simulink model "PD_double_pend"  (R2021a)
settings: Solver=FixedStepAuto  StartTime=0.0  StopTime=10  FixedStep=.01  RelTol=1e-3
model workspace (MAT data in the model file):
  exo_pos_cost_10 = param.Continuous
  exo_pos_cost_10.Size_ = [1 1]
  exo_pos_cost_10.Value_ = 1.48511326465
  exo_pos_cost_10.pID = paramid.Variable
  exo_pos_cost_10.pID.Name = 'exo_pos_cost'
values from neighbouring files (symbols this model uses):
  Dm1 = [1000,0;0,103.228187679703]    [no_exo.m]    (also in non_same_length.m = [30,0;0,30]; play_file.m = [30,0;0,30]; play_file22.m = [300,0;0,300]; play_file23.m = [30,0;0,30])
  Km1 = [1000,0;0,1000]    [no_exo.m]    (also in non_same_length.m = [30, 0; 0 30]; play_file.m = [30, 0; 0 30]; play_file22.m = [300, 0; 0 300]; play_file23.m = [30, 0; 0 30])
  l = [0.324, 0.3900]    [myStateTransitionFcn.m]
  lh = [0.324, 0.3900]    [no_exo.m]    (also in non_same_length.m; play_file.m; play_file22.m; play_file23.m)
  mh = [11.824, 3.848]    [no_exo.m]    (also in non_same_length.m; play_file.m; play_file22.m; play_file23.m)
undefined symbols (not defined in the file or in its folder): l1, l2, me2
libraries: robotcorelib x1
settings Model: Creator=nathanielgoldfarb  LastModifiedBy=nathanielgoldfarb
settings SolverCC: AlgebraicLoopSolver=TrustRegion
settings DataIOCC: ReturnWorkspaceOutputsName=SDOSimTest_Log
settings DebuggingCC: SFMachineParentedDataDiag=warning

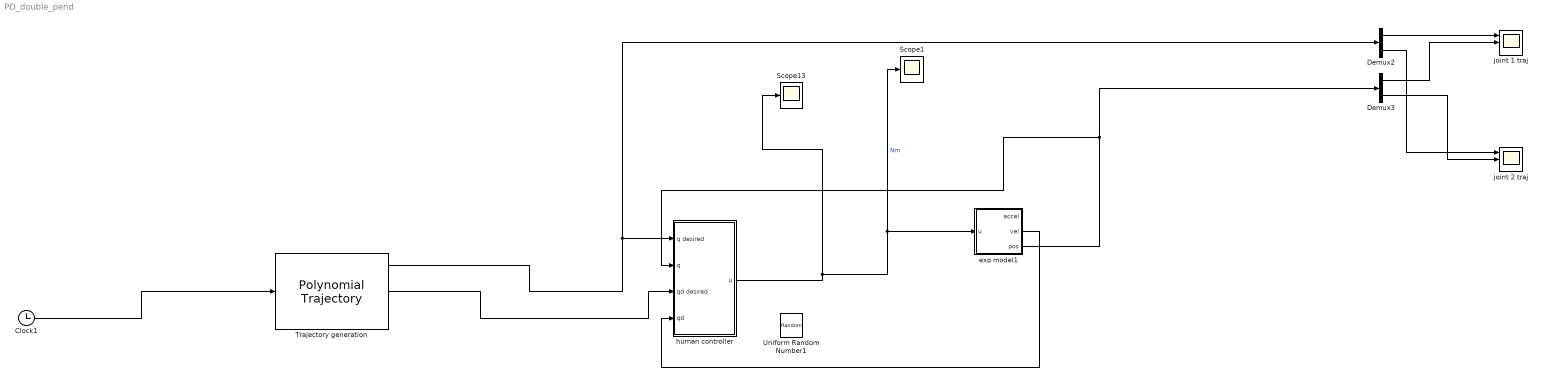
== system PD_double_pend ==
  Clock1 : Clock
  Demux2 : Demux  Outputs=2
  Demux3 : Demux  Outputs=2
  Scope1 : Scope
  Scope13 : Scope
  Trajectory generation : robotcorelib/Polynomial Trajectory  WaypointSource=Internal  Waypoints="[ 0 , -pi, 0;  0 -0.5*pi,0 ]"  TimePoints=[ 0, 5, 10]  TimeInterval=[ 1, 4 ]  Method=Cubic Polynomial  ParameterSource=Internal  VelocityBoundaryCondition=zeros( 2, 3 )  AccelerationBoundaryCondition=zeros( 2, 5 )  SimulateUsing=Interpreted execution
  Uniform Random Number1 : UniformRandomNumber  Minimum=-10  Maximum=10  SampleTime=0.1
  exo model1 : Subsystem
  human controller : Subsystem
  joint 1 traj : Scope  NumInputPorts=3
  joint 2 traj : Scope  NumInputPorts=3
  wires:
  Demux3/1 -> joint 1 traj/2
  Clock1/1 -> Trajectory generation/1
  Demux2/1 -> joint 1 traj/1
  Trajectory generation/1 -> human controller/1(q desired), Demux2/1
  Demux3/2 -> joint 2 traj/2
  Trajectory generation/2 -> human controller/3(qd desired)
  exo model1/3(pos) -> Demux3/1, human controller/2(q)
  exo model1/2(vel) -> human controller/4(qd)
  human controller/1(u) -> exo model1/1(u), Scope1/1, Scope13/1  "Nm"
  Demux2/2 -> joint 2 traj/1

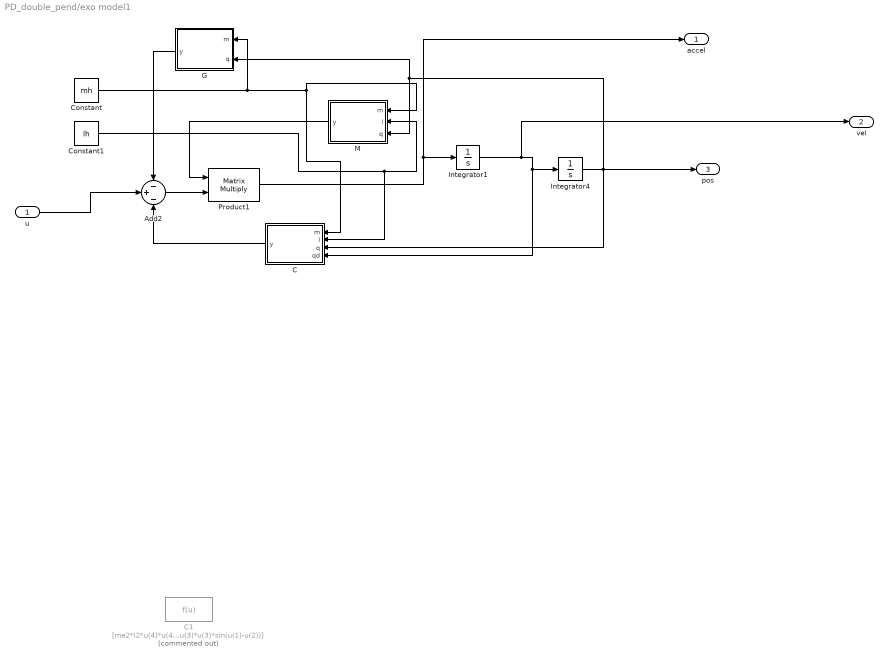
== system PD_double_pend/exo model1 ==
  u : Inport
  Add2 : Sum  Inputs=-+-
  C : MATLAB Function  TreatAsAtomicUnit=on
  C1 : Fcn  Commented=on  Expr=[me2*l2*u(4)*u(4)*sin(u(1)-u(2)); -me2*l1*u(3)*u(3)*sin(u(1)-u(2))]
  Constant : Constant  Value=mh
  Constant1 : Constant  Value=lh
  G : MATLAB Function  TreatAsAtomicUnit=on
  Integrator1 : Integrator  InitialCondition=[0;0]
  Integrator4 : Integrator  InitialCondition=[0.01;0.01]
  M : MATLAB Function  TreatAsAtomicUnit=on
  Product1 : Product  Multiplication=Matrix(*)
  accel : Outport
  vel : Outport  Port=2
  pos : Outport  Port=3
  wires:
  Constant/1 -> G/1(m), M/1(m), C/1(m)
  M/1(y) -> Product1/1
  Add2/1 -> Product1/2
  C/1(y) -> Add2/3
  G/1(y) -> Add2/1
  u/1 -> Add2/2
  Product1/1 -> accel/1, Integrator1/1
  Constant1/1 -> C/2(l), M/2(l)
  Integrator4/1 -> C/3(q), pos/1, M/3(q), G/2(q)
  Integrator1/1 -> vel/1, C/4(qd), Integrator4/1

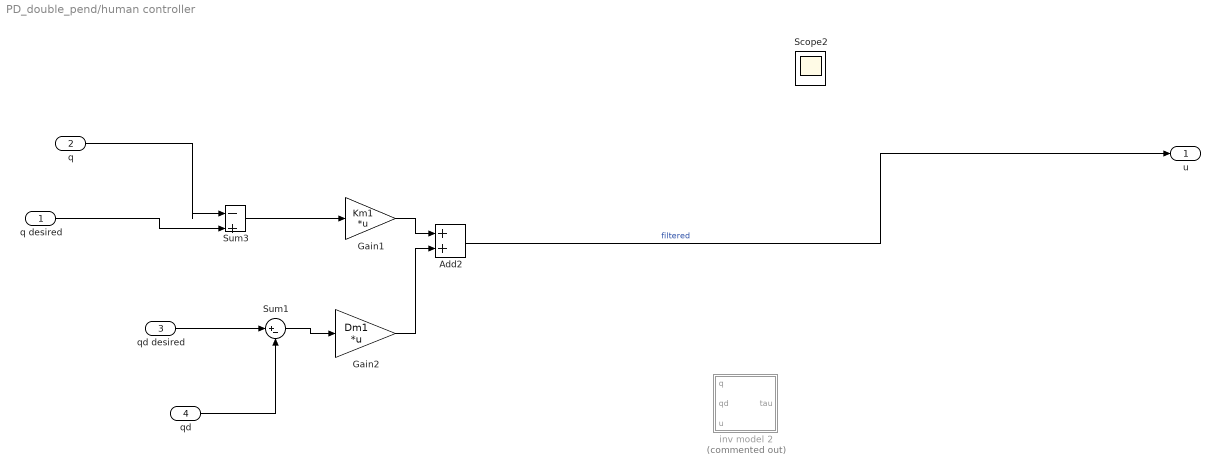
== system PD_double_pend/human controller ==
  q desired : Inport
  q : Inport  Port=2
  qd desired : Inport  Port=3
  qd : Inport  Port=4
  Add2 : Sum
  Gain1 : Gain  Gain=Km1  Multiplication=Matrix(K*u)
  Gain2 : Gain  Gain=Dm1  Multiplication=Matrix(K*u)
  Scope2 : Scope  NumInputPorts=3
  Sum1 : Sum  Inputs=|+-
  Sum3 : Sum  Inputs=|-+
  inv model 2 : Subsystem  Commented=on
  u : Outport
  wires:
  Sum1/1 -> Gain2/1
  qd/1 -> Sum1/2
  Sum3/1 -> Gain1/1
  Gain2/1 -> Add2/2
  q desired/1 -> Sum3/2
  Gain1/1 -> Add2/1
  qd desired/1 -> Sum1/1
  q/1 -> Sum3/1
  Add2/1 -> u/1  "filtered"

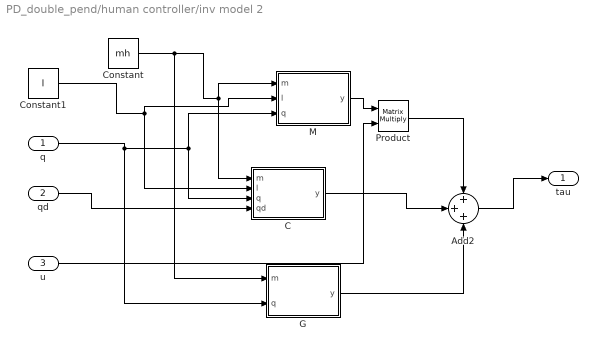
== system PD_double_pend/human controller/inv model 2 ==
  q : Inport
  qd : Inport  Port=2
  "u " : Inport  Port=3
  Add2 : Sum  Inputs=+++
  C : MATLAB Function  TreatAsAtomicUnit=on
  Constant : Constant  Value=mh
  Constant1 : Constant  Value=l
  G : MATLAB Function  TreatAsAtomicUnit=on
  M : MATLAB Function  TreatAsAtomicUnit=on
  Product : Product  Multiplication=Matrix(*)
  "tau " : Outport
  wires:
  Constant1/1 -> C/2(l), M/2(l)
  Constant/1 -> G/1(m), C/1(m), M/1(m)
  "u "/1 -> Product/2
  Product/1 -> Add2/1
  M/1(y) -> Product/1
  qd/1 -> C/4(qd)
  q/1 -> G/2(q), C/3(q), M/3(q)
  Add2/1 -> "tau "/1
  C/1(y) -> Add2/2
  G/1(y) -> Add2/3

== matlab function PD_double_pend/human controller/inv model 2/C ==
  data: m input; l input; q input; y output; qd input
function y = fcn(m, l, q, qd)



y = C(m, l, q, qd); % [m(2)*l(2)*qd(2)*qd(2)*sin(q(1)-q(2)); -m(2)*l(1)*qd(1)*qd(1)*sin(q(1)-q(2))];

== matlab function PD_double_pend/human controller/inv model 2/G ==
  data: m input; q input; y output
function y = fcn(m, q)
 y =  G(m,q);
end

== matlab function PD_double_pend/human controller/inv model 2/M ==
  data: m input; l input; q input; y output
function y = fcn(m, l, q)

y = M(m,l,q); % pinv([ (m(1)+m(2)) *l(1), m(2)*l(2)*cos(q(1)-q(2)); m(2)* l(1)*cos(q(1)-q(2)), m(2)*l(2)] );

end

== matlab function PD_double_pend/exo model1/C ==
  data: m input; l input; q input; y output; qd input
function y = fcn(m, l, q, qd)



y = C(m, l, q, qd); % [m(2)*l(2)*qd(2)*qd(2)*sin(q(1)-q(2)); -m(2)*l(1)*qd(1)*qd(1)*sin(q(1)-q(2))];

== matlab function PD_double_pend/exo model1/G ==
  data: m input; q input; y output
function y = fcn(m, q)
 y = [50; 50] + G(m,q);
end

== matlab function PD_double_pend/exo model1/M ==
  data: m input; l input; q input; y output
function y = fcn(m, l, q)

y = pinv(M(m,l,q)); % pinv([ (m(1)+m(2)) *l(1), m(2)*l(2)*cos(q(1)-q(2)); m(2)* l(1)*cos(q(1)-q(2)), m(2)*l(2)] );

end
